simulink model "Simple_Model_Packaging_7"  (R2024a)
settings: Solver=VariableStepAuto  StartTime=0.0  StopTime=0.004  RelTol=1e-3
InitFcn:
  | Parameter_Initialize_7
undefined symbols (not defined in the file or in its folder): b, gcbh, ISDFJ_parameter, magnitude, model, n, rcfiltgaincompat, Signal_delay_length, tao, Ts
libraries: simulink x9, commdigbbndfm2 x3, commsink2 x2, commdigbbndam3 x2, commfilt2 x2, commrandsrc3 x2, commchan3 x1, commrfcorlib x1, dspsigops x1, commdigbbndcpm2 x1, commseqgen3 x1, commutil2 x1
(part 2 of 2)

== matlab function Simple_Model_Packaging_7/MATLAB Function1 ==
  data: y output; t input; f input
% function y = carrierGenerator(t)
%     fc = 5e6;
%     y = exp(1i*2*pi*fc*t);

function y = carrierGenerator(t, f)
    y = exp(1i*2*pi*f*t);
end

== matlab function Simple_Model_Packaging_7/信道模型封装/NosieGen/调制方式/PM/MATLAB Function ==
  data: t input; signal input; y output; A input; freq input; K input; phi0 input
function y = PM(t, signal, A, freq, K, phi0)
   y = A*cos(2*pi*freq*t+K*signal+phi0) ;
end

== matlab function Simple_Model_Packaging_7/信道模型封装/NosieGen/多频干扰/MultiRandomFreq/MATLAB Function1 ==
  data: y output; t input; f input
% function y = carrierGenerator(t)
%     fc = 5e6;
%     y = exp(1i*2*pi*fc*t);

function y = carrierGenerator(t, f)
    y = exp(1i*2*pi*f*t);
end

== matlab function Simple_Model_Packaging_7/信道模型封装/NosieGen/多频干扰/MultiFreq/MultiFreqSignal ==
  data: y output; t input; MFF input; A input
function y  = MultiFreqSignal(t, MFF,A)
    % MFF表示输入的多频信号的频率与原信号的频率间隔
    % t表示采样时间
    % Signal表示需要被多频调制的原信号
    % A表示对应幅值
    % Phi0表示对应相位
    N = length(MFF); 
    MultitoneSignal =complex(zeros(N,1));
    for num1=1:N
        MultitoneSignal(num1) = A(num1).*exp(1j*(2*pi.*MFF(num1)*t));
    end
    y = sum(MultitoneSignal,"all");
end

== matlab function Simple_Model_Packaging_7/信道模型封装/NosieGen/多频干扰/MultiRandomFreq/MultiFreqSignal ==
  data: y output; t input; MFF input; A input
function y  = MultiFreqSignal(t, MFF,A)
    % MFF表示输入的多频信号的频率与原信号的频率间隔
    % t表示采样时间
    % Signal表示需要被多频调制的原信号
    % A表示对应幅值
    % Phi0表示对应相位
    N = length(MFF); 
    MultitoneSignal =complex(zeros(N,1));
    for num1=1:N
        MultitoneSignal(num1) = A(num1).*exp(1j*(2*pi.*MFF(num1)*t));
    end
    y = sum(MultitoneSignal,"all");
end

== matlab function Simple_Model_Packaging_7/信道模型封装/间歇转发干扰/MATLAB Function ==
  data: u input; y output; t input; Ts input; tau input; n input; buffer_size input; RandomPhaseFlag input; CodePeriod input
function y = isdfj_interference(u, t, Ts, tau, n, buffer_size, RandomPhaseFlag, CodePeriod)
% 输入：u(雷达信号), t(当前时间), params(干扰参数结构体)
% 输出：y(干扰信号)

persistent buffer last_sample_time sample_count;
persistent last_code_period_start current_phase;  % 新增持久变量

if isempty(buffer)
    buffer = complex(zeros(1, buffer_size));  % 初始化采样缓冲区
    last_sample_time = 0;
    sample_count = 0;
    last_code_period_start = -inf;  % 初始化码元周期起始时间
    current_phase = 1;             % 初始相位因子=1（无相位偏移）
end

% 1. 计算当前码元周期起始时间（关键修改）
current_period_start = floor(t / CodePeriod) * CodePeriod;

% 2. 若进入新码元周期，生成新随机相位
if current_period_start > last_code_period_start
    phi = round(2 * rand() - 1) * pi ;  % 生成[-π, π]的随机相位
    current_phase = exp(1i * phi);      % 复数相位因子
    last_code_period_start = current_period_start; % 更新周期标记
end

% 3. 采样阶段：在脉宽τ内捕获信号
if mod(t, Ts) < tau
    % 更新缓冲区（先进先出）
    buffer = [u, buffer(1:end-1)];  
    last_sample_time = t;
    sample_count = 0;  % 重置转发计数器
    y = complex(0);  % 采样阶段无输出
    
% 4. 转发阶段：重复转发n points
elseif (t - last_sample_time) <= n* tau && sample_count < n * buffer_size
    output_index = mod(sample_count, buffer_size);

    if RandomPhaseFlag == 0
        y = complex(buffer(end-output_index));  % 输出缓冲区值（fifo）
    else
        % 使用当前码元周期的相位因子（同一周期内不变）
        y = complex(buffer(end-output_index)) * current_phase; 
    end
    sample_count = sample_count + 1;

else
    y = complex(0);  % 非活跃期输出0
end
end

== matlab function Simple_Model_Packaging_7/信道模型封装/MATLAB Function1 ==
  data: u input; y output; t input; tau input; n input; buffer_size input
function y = isdfj_interference(u, t, tau, n, buffer_size)
% 输入：u(雷达信号), t(当前时间), params(干扰参数结构体)
% 输出：y(干扰信号)

persistent buffer last_sample_time sample_count Ts;
if isempty(buffer)
    buffer = complex(zeros(1, buffer_size));  % 初始化采样缓冲区
    last_sample_time = 0;
    sample_count = 0;
    Ts = tau * (n+1);
end

% 1. 采样阶段：在脉宽τ内捕获信号
if mod(t, Ts) < tau
    % 更新缓冲区（先进先出）
    buffer = [u, buffer(1:end-1)];  
    last_sample_time = t;
    sample_count = 0;  % 重置转发计数器
    y = complex(0);  % 采样阶段无输出
    
% 2. 转发阶段：重复转发n次
elseif (t - last_sample_time) >= tau && sample_count < n
    output_index = mod(sample_count, buffer_size);
    y = complex(buffer(end-output_index));  % 输出缓冲区值（fifo）
    sample_count = sample_count + 1;
else
    y = complex(0);  % 非活跃期输出0
end
end

== matlab function Simple_Model_Packaging_7/MATLAB Function ==
  data: y output; t input; f_chirp_min input; f_chirp_max input; T_chirp input
% function y = carrierGenerator(t)
%     fc = 5e6;
%     y = exp(1i*2*pi*fc*t);

function y = carrierGenerator(t, f_chirp_min, f_chirp_max, T_chirp)
    k_chirp = (f_chirp_max-f_chirp_min)/T_chirp;
    t = mod(t,T_chirp);
    y = exp(1i*2*pi*(f_chirp_min*t+0.5*k_chirp*t^2));

end

== matlab function Simple_Model_Packaging_7/信道模型封装/NosieGen/干扰方式/ChirpBasebandSignalGenerate/Chirp_Signal_Generation ==
  data: y output; t input; f_chirp_min input; T_chirp input; k_chirp input
function y = ChirpSignal(t, f_chirp_min, T_chirp, k_chirp)
    t = mod(t,T_chirp);
    y = exp(1i*2*pi*(f_chirp_min*t+0.5*k_chirp*t^2));
end

== matlab function Simple_Model_Packaging_7/信道模型封装/NosieGen/干扰源/Monophonic Sine Noise/Monophonic_Generate ==
  data: t input; A input; freq input; monophonic output; phi0 input
function monophonic = MonophonicGenerate(t, A, freq, phi0)
    monophonic = A * sin(2*pi*freq*t+phi0);
end

== matlab function Simple_Model_Packaging_7/信道模型封装/NosieGen/干扰源/Monophonic Sine Noise/Multitone_Interference_Generate ==
  data: SineNoiseFreqNum input; Multitone_interference output; SineNoiseFreq input; SineNoiseAmplitude input; t input
function Multitone_interference = fcn(SineNoiseFreqNum, SineNoiseFreq, SineNoiseAmplitude, t)
Multitone_interference = 0;

for index = 1:SineNoiseFreqNum
    Multitone_interference_subinterference = SineNoiseAmplitude(index) * sin(2*pi*SineNoiseFreq(index)*t);
    Multitone_interference = Multitone_interference + Multitone_interference_subinterference;
end

== matlab function Simple_Model_Packaging_7/rateTransitionUserDefined ==
  data: y output; input input
% function y = carrierGenerator(t)
%     fc = 5e6;
%     y = exp(1i*2*pi*fc*t);

function y = rateTransition(input)
    p = 1;
    q = 1;
    y = resample(input,p,q);
%     y(1:100) = repmat(y(100),1,100);
%     y(end-99:end) = repmat(y(end-99),1,100);
end

== matlab function Simple_Model_Packaging_7/MATLAB Function3 ==
  data: y output; input input
% function y = carrierGenerator(t)
%     fc = 5e6;
%     y = exp(1i*2*pi*fc*t);

function y = rateTransition(input)
    p = 1;
    q = 1;
    y = resample(input,p,q);
%     y(1:10) = repmat(y(10),1,10);
%     y(end-9:end) = repmat(y(end-9),1,10);
end

== matlab function Simple_Model_Packaging_7/信道模型封装/NosieGen/干扰源/Random Binary Noise/Random Binary Modulation ==
  data: Jn input; Jt output; t input; A input; freq input; phi0 input
function Jt = fcn(Jn,t,A,freq,phi0)
    Jt = A*Jn*cos(2*pi*freq*t+phi0);
end

== matlab function Simple_Model_Packaging_7/信道模型封装/NosieGen/干扰方式/StepSweepSignalGenerate/StepSweep_Signal ==
  data: y output; t input; f_stepSweep_min input; T_stepSweep input; delta_f_stepSweep input; T_stepSweep_dwell input; Ts input; N_stepSweep input
function y  = StepSweep(t, f_stepSweep_min, T_stepSweep, delta_f_stepSweep, T_stepSweep_dwell, Ts, N_stepSweep)
    % 时间，扫频最小值，扫频周期，单位扫频步进，扫频单位时间，噪声信号采样时间，扫频点数
    a = mod(t,T_stepSweep) + Ts/10000;
    b = fix(a/T_stepSweep_dwell);
    if b == N_stepSweep
        b = N_stepSweep - 1;
    end
    f = (f_stepSweep_min + b*delta_f_stepSweep);
    y = exp(1i*2*pi*f*t);
end

== matlab function Simple_Model_Packaging_7/信道模型封装/NosieGen/干扰源/PN MSK Noise/Random Binary Modulation ==
  data: cita_k input; MSKSignal output; t input; freq input
function MSKSignal = fcn(cita_k, t, freq)
    MSKSignal = cita_k * cos(2*pi*freq*t);
end
